simulink model "autopilot_altered"  (R2016a)
settings: Solver=FixedStepAuto  StartTime=0.0  StopTime=400  RelTol=1e-3
values from neighbouring files (symbols this model uses):
  U_trim = [0.0079    0.0000         0    0.1240]'    [run_auto_dubins.m]
  Vad = 18    [run_auto_dubins.m]
  X_trim = [0.0000    0.0000 -100.0000    0.9997    0.0000    0.0232   -0.0000 18.0168    0.0001    0.8366    0.0000    0.0000    0.0000 0.0039 -0.0000    0.0039   -0.0000    0.1240]'    [run_auto_dubins.m]
undefined symbols (not defined in the file or in its folder): p_nd
libraries: X8_lib x2, simulink x1
settings Model: Creator=andreanv  LastModifiedBy=andreanv

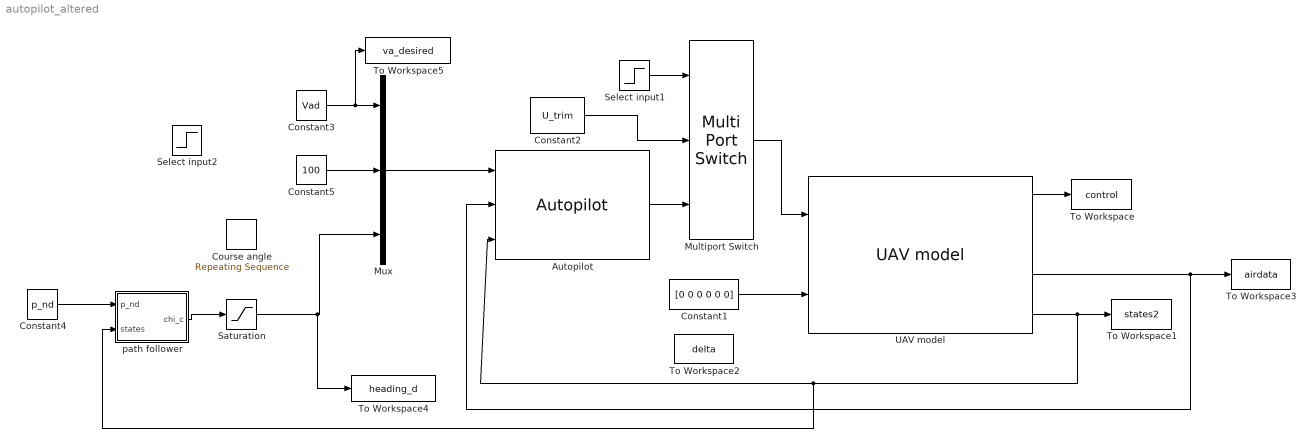
== system autopilot_altered ==
  Autopilot : X8_lib/Autopilot  param=param  X_trim=X_trim  U_trim=U_trim
  Constant1 : Constant  Value=[0 0 0 0 0 0]
  Constant2 : Constant  Value=U_trim
  Constant3 : Constant  Value=Vad
  Constant4 : Constant  Value=p_nd
  Constant5 : Constant  Value=100
  Course angle : simulink/Sources/Repeating Sequence  rep_seq_t=[0 5 30 31 50 65 100]  rep_seq_y=[0 pi/4 pi/4 pi/2 pi/2 pi/4 pi/4]
  Multiport Switch : MultiPortSwitch  Inputs=2
  Mux : Mux  Inputs=3
  Saturation : Saturate  UpperLimit=pi-0.04  LowerLimit=-pi+0.04
  Select input1 : Step  Before=1  After=2  SampleTime=0
  Select input2 : Step  After=-pi/4  SampleTime=0
  To Workspace : ToWorkspace  VariableName=control  SaveFormat=Timeseries  SampleTime=-1
  To Workspace1 : ToWorkspace  VariableName=states2  SaveFormat=Timeseries  SampleTime=-1
  To Workspace2 : ToWorkspace  VariableName=delta  SaveFormat=Timeseries  SampleTime=-1
  To Workspace3 : ToWorkspace  VariableName=airdata  SaveFormat=Timeseries  SampleTime=-1
  To Workspace4 : ToWorkspace  VariableName=heading_d  SaveFormat=Timeseries  SampleTime=-1
  To Workspace5 : ToWorkspace  VariableName=va_desired  SaveFormat=Timeseries  SampleTime=-1
  UAV model : X8_lib/UAV model  param=param  pos0=X_trim(1:3)'  quat0=X_trim(4:7)'  vel0=X_trim(8:10)'  rate0=X_trim(11:13)'  servoR_pos0=X_trim(14)'  servoR_vel0=X_trim(15)'  servoL_pos0=X_trim(16)'  servoL_vel0=X_trim(17)'  motor_speed0=X_trim(18)'
  path follower : MATLAB Function  TreatAsAtomicUnit=on
      mask init:
      | path = load('test.mat', 'p_nd');
  wires:
  Constant1/1 -> UAV model/2
  UAV model/4 -> path follower/2(states), Autopilot/3, To Workspace1/1
  Select input1/1 -> Multiport Switch/1
  UAV model/3 -> Autopilot/2, To Workspace3/1
  Mux/1 -> Autopilot/1
  Constant5/1 -> Mux/2
  Constant2/1 -> Multiport Switch/2
  Multiport Switch/1 -> UAV model/1
  UAV model/1 -> To Workspace/1
  Constant3/1 -> To Workspace5/1, Mux/1
  path follower/1(chi_c) -> Saturation/1
  Autopilot/1 -> Multiport Switch/3
  Saturation/1 -> To Workspace4/1, Mux/3
  Constant4/1 -> path follower/1(p_nd)

== matlab function autopilot_altered/path follower ==
  data: p_nd input; states input; chi_c output
function chi_c = fcn(p_nd, states)
%#codegen

chi_c = lineOfSight([states.Position.p_N, states.Position.p_E], p_nd);
